simulink model "RALFCANread_18b"  (R2018b)
settings: Solver=FixedStepAuto  StartTime=0.0  StopTime=inf  FixedStep=0.001  RelTol=1e-3
model workspace (MAT data in the model file):
  SL_ROS_VariableLengthArrays_MaxSizes.CommonInfo.ArrayTruncateAction = 'EmitWarning'
  SL_ROS_VariableLengthArrays_MaxSizes.MsgTypeMap = containers.Map
  SL_ROS_VariableLengthArrays_MaxSizes.MsgTypeMap.serialization.keys = {'std_msgs/Int16MultiArray'}
  SL_ROS_VariableLengthArrays_MaxSizes.MsgTypeMap.serialization.values{1}.PropertyName = 'Data'
  SL_ROS_VariableLengthArrays_MaxSizes.MsgTypeMap.serialization.values{1}.DataType = 'int16'
  SL_ROS_VariableLengthArrays_MaxSizes.MsgTypeMap.serialization.values{1}.MaxLength = 4
  SL_ROS_VariableLengthArrays_MaxSizes.MsgTypeMap.serialization.uniformity = 0
  SL_ROS_VariableLengthArrays_MaxSizes.MsgTypeMap.serialization.keyType = 'char'
  SL_ROS_VariableLengthArrays_MaxSizes.MsgTypeMap.serialization.valueType = 'any'
undefined symbols (not defined in the file): canChannel, Data, Data_SL_Info
libraries: etargetslib x4, canmsglib x4, robotlib x2, canlib x2
settings Model: Creator=alf  LastModifiedBy=giull
settings SFSimCC: SimUseLocalCustomCode=off
settings RTWCC: RTWUseLocalCustomCode=off

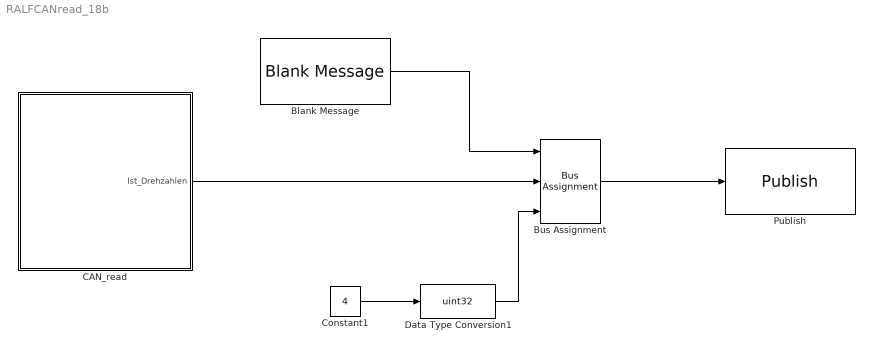
== system RALFCANread_18b ==
  Blank Message : robotlib/Blank Message  messageClass=Message  entityType=std_msgs/Int16MultiArray  messageType=std_msgs/Int16MultiArray  SampleTime=inf
      settings: SourceProductBaseCode=RO
  Bus Assignment : BusAssignment  AssignedSignals=Data,Data_SL_Info.CurrentLength
  CAN_read : Subsystem
  Constant1 : Constant  Value=4
  Data Type Conversion1 : DataTypeConversion  OutDataTypeStr=uint32
  Publish : robotlib/Publish  topicSource=Specify your own  topic=/CANread  messageType=std_msgs/Int16MultiArray  messageQueueLength=1
      settings: SourceProductBaseCode=RO
  wires:
  Constant1/1 -> Data Type Conversion1/1
  Data Type Conversion1/1 -> Bus Assignment/3
  Blank Message/1 -> Bus Assignment/1
  Bus Assignment/1 -> Publish/1
  CAN_read/1(Ist_Drehzahlen) -> Bus Assignment/2

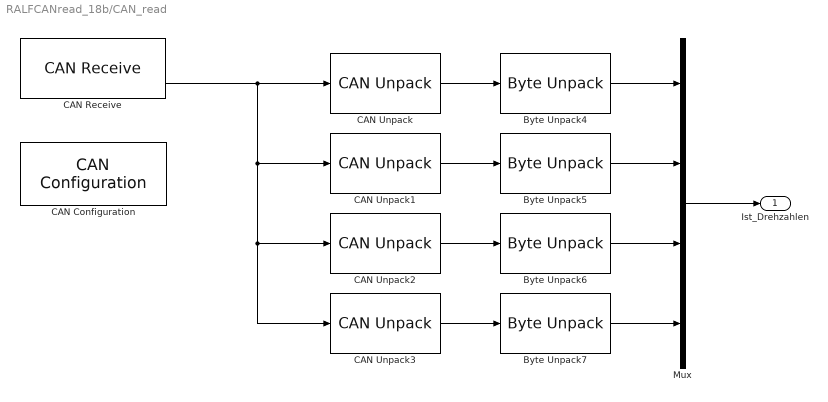
== system RALFCANread_18b/CAN_read ==
  Byte Unpack{4..7} (4 alike) : etargetslib/Byte Unpack  dimensions={[1]}  datatypes={'int16'}  byteAlign=1
      settings: SourceProductName=MATLAB Coder
  CAN Configuration : canlib/CAN Configuration  BlockHandle=9.0006  Device=MathWorks Virtual 1 (Channel 1)  DeviceMenu=MathWorks Virtual 1 (Channel 1)  ObjConstructor=canChannel('MathWorks', 'Virtual 1', 1)  BusSpeed=500000  EnableBitParameters=off  AckMode=Normal
      settings: SourceProductName=Vehicle Network Toolbox  SourceProductBaseCode=VN
  CAN Receive : canlib/CAN Receive  BlockHandle=10.0006  Device=MathWorks Virtual 1 (Channel 1)  DeviceMenu=MathWorks Virtual 1 (Channel 1)  ObjConstructor=canChannel('MathWorks', 'Virtual 1', 1)  EnableStandardIDsFilter=off  StdIDsCombo=Allow all  StandardIDs=0  EnableExtendedIDsFilter=off  ExtIDsCombo=Allow all  ExtendedIDs=0  SampleTime=0.01  MsgsPerTimestep=all  InternalFilterUpdateStatus=on  BusOutput=off
      settings: SourceProductName=Vehicle Network Toolbox  SourceProductBaseCode=VN
  CAN Unpack : canmsglib/CAN Unpack  MsgList=(none)  MsgName=CAN Msg  MsgIDType=Standard (11-bit identifier)  MsgIdentifier=259  MsgLength=8  IDPort=off  TimestampPort=off  ErrorPort=off  RemotePort=off  LengthPort=off  StatusPort=off  ApplyMinMax=off  NSignals=0  StartBits=0  SignalSizes=0  ByteOrders=0  DataTypes=0  MultiplexTypes=0  MultiplexValues=0  Factors=0  Offsets=0  Minimums=0  Maximums=0
      settings: SourceProductName=Vehicle Network Toolbox  SourceProductBaseCode=VN  DataFormat=raw data
  CAN Unpack1 : canmsglib/CAN Unpack  MsgList=(none)  MsgName=CAN Msg  MsgIDType=Standard (11-bit identifier)  MsgIdentifier=275  MsgLength=8  IDPort=off  TimestampPort=off  ErrorPort=off  RemotePort=off  LengthPort=off  StatusPort=off  ApplyMinMax=off  NSignals=0  StartBits=0  SignalSizes=0  ByteOrders=0  DataTypes=0  MultiplexTypes=0  MultiplexValues=0  Factors=0  Offsets=0  Minimums=0  Maximums=0
      settings: SourceProductName=Vehicle Network Toolbox  SourceProductBaseCode=VN  DataFormat=raw data
  CAN Unpack2 : canmsglib/CAN Unpack  MsgList=(none)  MsgName=CAN Msg  MsgIDType=Standard (11-bit identifier)  MsgIdentifier=291  MsgLength=8  IDPort=off  TimestampPort=off  ErrorPort=off  RemotePort=off  LengthPort=off  StatusPort=off  ApplyMinMax=off  NSignals=0  StartBits=0  SignalSizes=0  ByteOrders=0  DataTypes=0  MultiplexTypes=0  MultiplexValues=0  Factors=0  Offsets=0  Minimums=0  Maximums=0
      settings: SourceProductName=Vehicle Network Toolbox  SourceProductBaseCode=VN  DataFormat=raw data
  CAN Unpack3 : canmsglib/CAN Unpack  MsgList=(none)  MsgName=CAN Msg  MsgIDType=Standard (11-bit identifier)  MsgIdentifier=307  MsgLength=8  IDPort=off  TimestampPort=off  ErrorPort=off  RemotePort=off  LengthPort=off  StatusPort=off  ApplyMinMax=off  NSignals=0  StartBits=0  SignalSizes=0  ByteOrders=0  DataTypes=0  MultiplexTypes=0  MultiplexValues=0  Factors=0  Offsets=0  Minimums=0  Maximums=0
      settings: SourceProductName=Vehicle Network Toolbox  SourceProductBaseCode=VN  DataFormat=raw data
  Mux : Mux
  Ist_Drehzahlen : Outport  VectorParamsAs1DForOutWhenUnconnected=off
  wires:
  CAN Unpack/1 -> Byte Unpack4/1
  CAN Unpack2/1 -> Byte Unpack6/1
  CAN Unpack1/1 -> Byte Unpack5/1
  CAN Unpack3/1 -> Byte Unpack7/1
  Byte Unpack5/1 -> Mux/2
  Byte Unpack6/1 -> Mux/3
  Mux/1 -> Ist_Drehzahlen/1
  CAN Receive/2 -> CAN Unpack3/1, CAN Unpack2/1, CAN Unpack1/1, CAN Unpack/1
  Byte Unpack7/1 -> Mux/4
  Byte Unpack4/1 -> Mux/1
